simulink model "XMC_FFT2D_HDL_AIE"  (R2021a)
settings: Solver=FixedStepDiscrete  StartTime=0.0  StopTime=256*256*2  RelTol=1e-3
PreLoadFcn:
  | MRIDemo_PreloadFcn;
  | 
  | % configure hardware specifics information
  | clock_frequency = 150e6;
  | 
  | % corner bender info
  | clk = clock_frequency; %Hz
  | Tclk = 1/clk;
  | L2M = 8; % L2M=log2(M)
  | L2N = 8; % L2N=log2(N)
  | M = 2^L2M;
  | N = 2^L2N;
  | SSR = 1;
InitFcn:
  | xlEvaluateHDLBlocks('XMC_FFT2D_HDL_AIE')
undefined symbols (not defined in the file): c, gray, S, vsva2197, xcvc1902
libraries: hdlBasic x138, aieUtilities x3, dspxfrm3 x2, dspsrcs4 x2, aieDSP x2, simulink x1, vmcUtilities x1
(part 2 of 2)

== system XMC_FFT2D_HDL_AIE/hdl_corner_turn/Read BarrelShifter/RotateLeft5 ==
  I : Inport
  Concat : hdlBasic/Concat  num_inputs=2  XmcBlockStatus=1  maskContainerNames=group1  block_type=concat  block_config=sysgen:Concat_config
  Slice : hdlBasic/Slice  nbits=NB  boolean_output=off  mode=Upper Bit Location + Width  bit1=0  base1=MSB of Input  bit0=0  base0=LSB of Input  XmcBlockStatus=1  maskContainerNames=group1  block_type=slice  block_config=sysgen:Slice_config
  Slice1 : hdlBasic/Slice  nbits=W-NB  boolean_output=off  mode=Lower Bit Location + Width  bit1=0  base1=MSB of Input  bit0=0  base0=LSB of Input  XmcBlockStatus=1  maskContainerNames=group1  block_type=slice  block_config=sysgen:Slice_config
  O : Outport
  wires:
  I/1 -> Slice1/1, Slice/1
  Concat/1 -> O/1
  Slice/1 -> Concat/2
  Slice1/1 -> Concat/1

== system XMC_FFT2D_HDL_AIE/hdl_corner_turn/Read BarrelShifter/RotateLeft6 ==
  I : Inport
  Concat : hdlBasic/Concat  num_inputs=2  XmcBlockStatus=1  maskContainerNames=group1  block_type=concat  block_config=sysgen:Concat_config
  Slice : hdlBasic/Slice  nbits=NB  boolean_output=off  mode=Upper Bit Location + Width  bit1=0  base1=MSB of Input  bit0=0  base0=LSB of Input  XmcBlockStatus=1  maskContainerNames=group1  block_type=slice  block_config=sysgen:Slice_config
  Slice1 : hdlBasic/Slice  nbits=W-NB  boolean_output=off  mode=Lower Bit Location + Width  bit1=0  base1=MSB of Input  bit0=0  base0=LSB of Input  XmcBlockStatus=1  maskContainerNames=group1  block_type=slice  block_config=sysgen:Slice_config
  O : Outport
  wires:
  I/1 -> Slice1/1, Slice/1
  Concat/1 -> O/1
  Slice/1 -> Concat/2
  Slice1/1 -> Concat/1

== system XMC_FFT2D_HDL_AIE/hdl_corner_turn/Read BarrelShifter/RotateLeft7 ==
  I : Inport
  Concat : hdlBasic/Concat  num_inputs=2  XmcBlockStatus=1  maskContainerNames=group1  block_type=concat  block_config=sysgen:Concat_config
  Slice : hdlBasic/Slice  nbits=NB  boolean_output=off  mode=Upper Bit Location + Width  bit1=0  base1=MSB of Input  bit0=0  base0=LSB of Input  XmcBlockStatus=1  maskContainerNames=group1  block_type=slice  block_config=sysgen:Slice_config
  Slice1 : hdlBasic/Slice  nbits=W-NB  boolean_output=off  mode=Lower Bit Location + Width  bit1=0  base1=MSB of Input  bit0=0  base0=LSB of Input  XmcBlockStatus=1  maskContainerNames=group1  block_type=slice  block_config=sysgen:Slice_config
  O : Outport
  wires:
  I/1 -> Slice1/1, Slice/1
  Concat/1 -> O/1
  Slice/1 -> Concat/2
  Slice1/1 -> Concat/1

== system XMC_FFT2D_HDL_AIE/hdl_corner_turn/Read BarrelShifter/RotateLeft8 ==
  I : Inport
  Concat : hdlBasic/Concat  num_inputs=2  XmcBlockStatus=1  maskContainerNames=group1  block_type=concat  block_config=sysgen:Concat_config
  Slice : hdlBasic/Slice  nbits=NB  boolean_output=off  mode=Upper Bit Location + Width  bit1=0  base1=MSB of Input  bit0=0  base0=LSB of Input  XmcBlockStatus=1  maskContainerNames=group1  block_type=slice  block_config=sysgen:Slice_config
  Slice1 : hdlBasic/Slice  nbits=W-NB  boolean_output=off  mode=Lower Bit Location + Width  bit1=0  base1=MSB of Input  bit0=0  base0=LSB of Input  XmcBlockStatus=1  maskContainerNames=group1  block_type=slice  block_config=sysgen:Slice_config
  O : Outport
  wires:
  I/1 -> Slice1/1, Slice/1
  Concat/1 -> O/1
  Slice/1 -> Concat/2
  Slice1/1 -> Concat/1

== system XMC_FFT2D_HDL_AIE/hdl_corner_turn/Read BarrelShifter/RotateLeft9 ==
  I : Inport
  Concat : hdlBasic/Concat  num_inputs=2  XmcBlockStatus=1  maskContainerNames=group1  block_type=concat  block_config=sysgen:Concat_config
  Slice : hdlBasic/Slice  nbits=NB  boolean_output=off  mode=Upper Bit Location + Width  bit1=0  base1=MSB of Input  bit0=0  base0=LSB of Input  XmcBlockStatus=1  maskContainerNames=group1  block_type=slice  block_config=sysgen:Slice_config
  Slice1 : hdlBasic/Slice  nbits=W-NB  boolean_output=off  mode=Lower Bit Location + Width  bit1=0  base1=MSB of Input  bit0=0  base0=LSB of Input  XmcBlockStatus=1  maskContainerNames=group1  block_type=slice  block_config=sysgen:Slice_config
  O : Outport
  wires:
  I/1 -> Slice1/1, Slice/1
  Concat/1 -> O/1
  Slice/1 -> Concat/2
  Slice1/1 -> Concat/1

== system XMC_FFT2D_HDL_AIE/hdl_corner_turn/Write BarrelShifter/RotateLeft1 ==
  I : Inport
  Concat : hdlBasic/Concat  num_inputs=2  XmcBlockStatus=1  maskContainerNames=group1  block_type=concat  block_config=sysgen:Concat_config
  Slice : hdlBasic/Slice  nbits=NB  boolean_output=off  mode=Upper Bit Location + Width  bit1=0  base1=MSB of Input  bit0=0  base0=LSB of Input  XmcBlockStatus=1  maskContainerNames=group1  block_type=slice  block_config=sysgen:Slice_config
  Slice1 : hdlBasic/Slice  nbits=W-NB  boolean_output=off  mode=Lower Bit Location + Width  bit1=0  base1=MSB of Input  bit0=0  base0=LSB of Input  XmcBlockStatus=1  maskContainerNames=group1  block_type=slice  block_config=sysgen:Slice_config
  O : Outport
  wires:
  I/1 -> Slice1/1, Slice/1
  Concat/1 -> O/1
  Slice/1 -> Concat/2
  Slice1/1 -> Concat/1

== system XMC_FFT2D_HDL_AIE/hdl_corner_turn/Write BarrelShifter/RotateLeft10 ==
  I : Inport
  Concat : hdlBasic/Concat  num_inputs=2  XmcBlockStatus=1  maskContainerNames=group1  block_type=concat  block_config=sysgen:Concat_config
  Slice : hdlBasic/Slice  nbits=NB  boolean_output=off  mode=Upper Bit Location + Width  bit1=0  base1=MSB of Input  bit0=0  base0=LSB of Input  XmcBlockStatus=1  maskContainerNames=group1  block_type=slice  block_config=sysgen:Slice_config
  Slice1 : hdlBasic/Slice  nbits=W-NB  boolean_output=off  mode=Lower Bit Location + Width  bit1=0  base1=MSB of Input  bit0=0  base0=LSB of Input  XmcBlockStatus=1  maskContainerNames=group1  block_type=slice  block_config=sysgen:Slice_config
  O : Outport
  wires:
  Slice1/1 -> Concat/1
  Slice/1 -> Concat/2
  Concat/1 -> O/1
  I/1 -> Slice/1, Slice1/1

== system XMC_FFT2D_HDL_AIE/hdl_corner_turn/Write BarrelShifter/RotateLeft11 ==
  I : Inport
  Concat : hdlBasic/Concat  num_inputs=2  XmcBlockStatus=1  maskContainerNames=group1  block_type=concat  block_config=sysgen:Concat_config
  Slice : hdlBasic/Slice  nbits=NB  boolean_output=off  mode=Upper Bit Location + Width  bit1=0  base1=MSB of Input  bit0=0  base0=LSB of Input  XmcBlockStatus=1  maskContainerNames=group1  block_type=slice  block_config=sysgen:Slice_config
  Slice1 : hdlBasic/Slice  nbits=W-NB  boolean_output=off  mode=Lower Bit Location + Width  bit1=0  base1=MSB of Input  bit0=0  base0=LSB of Input  XmcBlockStatus=1  maskContainerNames=group1  block_type=slice  block_config=sysgen:Slice_config
  O : Outport
  wires:
  Slice1/1 -> Concat/1
  Slice/1 -> Concat/2
  Concat/1 -> O/1
  I/1 -> Slice/1, Slice1/1

== system XMC_FFT2D_HDL_AIE/hdl_corner_turn/Write BarrelShifter/RotateLeft12 ==
  I : Inport
  Concat : hdlBasic/Concat  num_inputs=2  XmcBlockStatus=1  maskContainerNames=group1  block_type=concat  block_config=sysgen:Concat_config
  Slice : hdlBasic/Slice  nbits=NB  boolean_output=off  mode=Upper Bit Location + Width  bit1=0  base1=MSB of Input  bit0=0  base0=LSB of Input  XmcBlockStatus=1  maskContainerNames=group1  block_type=slice  block_config=sysgen:Slice_config
  Slice1 : hdlBasic/Slice  nbits=W-NB  boolean_output=off  mode=Lower Bit Location + Width  bit1=0  base1=MSB of Input  bit0=0  base0=LSB of Input  XmcBlockStatus=1  maskContainerNames=group1  block_type=slice  block_config=sysgen:Slice_config
  O : Outport
  wires:
  Slice1/1 -> Concat/1
  Slice/1 -> Concat/2
  Concat/1 -> O/1
  I/1 -> Slice/1, Slice1/1

== system XMC_FFT2D_HDL_AIE/hdl_corner_turn/Write BarrelShifter/RotateLeft13 ==
  I : Inport
  Concat : hdlBasic/Concat  num_inputs=2  XmcBlockStatus=1  maskContainerNames=group1  block_type=concat  block_config=sysgen:Concat_config
  Slice : hdlBasic/Slice  nbits=NB  boolean_output=off  mode=Upper Bit Location + Width  bit1=0  base1=MSB of Input  bit0=0  base0=LSB of Input  XmcBlockStatus=1  maskContainerNames=group1  block_type=slice  block_config=sysgen:Slice_config
  Slice1 : hdlBasic/Slice  nbits=W-NB  boolean_output=off  mode=Lower Bit Location + Width  bit1=0  base1=MSB of Input  bit0=0  base0=LSB of Input  XmcBlockStatus=1  maskContainerNames=group1  block_type=slice  block_config=sysgen:Slice_config
  O : Outport
  wires:
  Slice1/1 -> Concat/1
  Slice/1 -> Concat/2
  Concat/1 -> O/1
  I/1 -> Slice/1, Slice1/1

== system XMC_FFT2D_HDL_AIE/hdl_corner_turn/Write BarrelShifter/RotateLeft14 ==
  I : Inport
  Concat : hdlBasic/Concat  num_inputs=2  XmcBlockStatus=1  maskContainerNames=group1  block_type=concat  block_config=sysgen:Concat_config
  Slice : hdlBasic/Slice  nbits=NB  boolean_output=off  mode=Upper Bit Location + Width  bit1=0  base1=MSB of Input  bit0=0  base0=LSB of Input  XmcBlockStatus=1  maskContainerNames=group1  block_type=slice  block_config=sysgen:Slice_config
  Slice1 : hdlBasic/Slice  nbits=W-NB  boolean_output=off  mode=Lower Bit Location + Width  bit1=0  base1=MSB of Input  bit0=0  base0=LSB of Input  XmcBlockStatus=1  maskContainerNames=group1  block_type=slice  block_config=sysgen:Slice_config
  O : Outport
  wires:
  Slice1/1 -> Concat/1
  Slice/1 -> Concat/2
  Concat/1 -> O/1
  I/1 -> Slice/1, Slice1/1

== system XMC_FFT2D_HDL_AIE/hdl_corner_turn/Write BarrelShifter/RotateLeft15 ==
  I : Inport
  Concat : hdlBasic/Concat  num_inputs=2  XmcBlockStatus=1  maskContainerNames=group1  block_type=concat  block_config=sysgen:Concat_config
  Slice : hdlBasic/Slice  nbits=NB  boolean_output=off  mode=Upper Bit Location + Width  bit1=0  base1=MSB of Input  bit0=0  base0=LSB of Input  XmcBlockStatus=1  maskContainerNames=group1  block_type=slice  block_config=sysgen:Slice_config
  Slice1 : hdlBasic/Slice  nbits=W-NB  boolean_output=off  mode=Lower Bit Location + Width  bit1=0  base1=MSB of Input  bit0=0  base0=LSB of Input  XmcBlockStatus=1  maskContainerNames=group1  block_type=slice  block_config=sysgen:Slice_config
  O : Outport
  wires:
  Slice1/1 -> Concat/1
  Slice/1 -> Concat/2
  Concat/1 -> O/1
  I/1 -> Slice/1, Slice1/1

== system XMC_FFT2D_HDL_AIE/hdl_corner_turn/Write BarrelShifter/RotateLeft2 ==
  I : Inport
  Concat : hdlBasic/Concat  num_inputs=2  XmcBlockStatus=1  maskContainerNames=group1  block_type=concat  block_config=sysgen:Concat_config
  Slice : hdlBasic/Slice  nbits=NB  boolean_output=off  mode=Upper Bit Location + Width  bit1=0  base1=MSB of Input  bit0=0  base0=LSB of Input  XmcBlockStatus=1  maskContainerNames=group1  block_type=slice  block_config=sysgen:Slice_config
  Slice1 : hdlBasic/Slice  nbits=W-NB  boolean_output=off  mode=Lower Bit Location + Width  bit1=0  base1=MSB of Input  bit0=0  base0=LSB of Input  XmcBlockStatus=1  maskContainerNames=group1  block_type=slice  block_config=sysgen:Slice_config
  O : Outport
  wires:
  Slice1/1 -> Concat/1
  Slice/1 -> Concat/2
  Concat/1 -> O/1
  I/1 -> Slice/1, Slice1/1

== system XMC_FFT2D_HDL_AIE/hdl_corner_turn/Write BarrelShifter/RotateLeft3 ==
  I : Inport
  Concat : hdlBasic/Concat  num_inputs=2  XmcBlockStatus=1  maskContainerNames=group1  block_type=concat  block_config=sysgen:Concat_config
  Slice : hdlBasic/Slice  nbits=NB  boolean_output=off  mode=Upper Bit Location + Width  bit1=0  base1=MSB of Input  bit0=0  base0=LSB of Input  XmcBlockStatus=1  maskContainerNames=group1  block_type=slice  block_config=sysgen:Slice_config
  Slice1 : hdlBasic/Slice  nbits=W-NB  boolean_output=off  mode=Lower Bit Location + Width  bit1=0  base1=MSB of Input  bit0=0  base0=LSB of Input  XmcBlockStatus=1  maskContainerNames=group1  block_type=slice  block_config=sysgen:Slice_config
  O : Outport
  wires:
  Slice1/1 -> Concat/1
  Slice/1 -> Concat/2
  Concat/1 -> O/1
  I/1 -> Slice/1, Slice1/1

== system XMC_FFT2D_HDL_AIE/hdl_corner_turn/Write BarrelShifter/RotateLeft4 ==
  I : Inport
  Concat : hdlBasic/Concat  num_inputs=2  XmcBlockStatus=1  maskContainerNames=group1  block_type=concat  block_config=sysgen:Concat_config
  Slice : hdlBasic/Slice  nbits=NB  boolean_output=off  mode=Upper Bit Location + Width  bit1=0  base1=MSB of Input  bit0=0  base0=LSB of Input  XmcBlockStatus=1  maskContainerNames=group1  block_type=slice  block_config=sysgen:Slice_config
  Slice1 : hdlBasic/Slice  nbits=W-NB  boolean_output=off  mode=Lower Bit Location + Width  bit1=0  base1=MSB of Input  bit0=0  base0=LSB of Input  XmcBlockStatus=1  maskContainerNames=group1  block_type=slice  block_config=sysgen:Slice_config
  O : Outport
  wires:
  Slice1/1 -> Concat/1
  Slice/1 -> Concat/2
  Concat/1 -> O/1
  I/1 -> Slice/1, Slice1/1

== system XMC_FFT2D_HDL_AIE/hdl_corner_turn/Write BarrelShifter/RotateLeft5 ==
  I : Inport
  Concat : hdlBasic/Concat  num_inputs=2  XmcBlockStatus=1  maskContainerNames=group1  block_type=concat  block_config=sysgen:Concat_config
  Slice : hdlBasic/Slice  nbits=NB  boolean_output=off  mode=Upper Bit Location + Width  bit1=0  base1=MSB of Input  bit0=0  base0=LSB of Input  XmcBlockStatus=1  maskContainerNames=group1  block_type=slice  block_config=sysgen:Slice_config
  Slice1 : hdlBasic/Slice  nbits=W-NB  boolean_output=off  mode=Lower Bit Location + Width  bit1=0  base1=MSB of Input  bit0=0  base0=LSB of Input  XmcBlockStatus=1  maskContainerNames=group1  block_type=slice  block_config=sysgen:Slice_config
  O : Outport
  wires:
  Slice1/1 -> Concat/1
  Slice/1 -> Concat/2
  Concat/1 -> O/1
  I/1 -> Slice/1, Slice1/1

== system XMC_FFT2D_HDL_AIE/hdl_corner_turn/Write BarrelShifter/RotateLeft6 ==
  I : Inport
  Concat : hdlBasic/Concat  num_inputs=2  XmcBlockStatus=1  maskContainerNames=group1  block_type=concat  block_config=sysgen:Concat_config
  Slice : hdlBasic/Slice  nbits=NB  boolean_output=off  mode=Upper Bit Location + Width  bit1=0  base1=MSB of Input  bit0=0  base0=LSB of Input  XmcBlockStatus=1  maskContainerNames=group1  block_type=slice  block_config=sysgen:Slice_config
  Slice1 : hdlBasic/Slice  nbits=W-NB  boolean_output=off  mode=Lower Bit Location + Width  bit1=0  base1=MSB of Input  bit0=0  base0=LSB of Input  XmcBlockStatus=1  maskContainerNames=group1  block_type=slice  block_config=sysgen:Slice_config
  O : Outport
  wires:
  Slice1/1 -> Concat/1
  Slice/1 -> Concat/2
  Concat/1 -> O/1
  I/1 -> Slice/1, Slice1/1

== system XMC_FFT2D_HDL_AIE/hdl_corner_turn/Write BarrelShifter/RotateLeft7 ==
  I : Inport
  Concat : hdlBasic/Concat  num_inputs=2  XmcBlockStatus=1  maskContainerNames=group1  block_type=concat  block_config=sysgen:Concat_config
  Slice : hdlBasic/Slice  nbits=NB  boolean_output=off  mode=Upper Bit Location + Width  bit1=0  base1=MSB of Input  bit0=0  base0=LSB of Input  XmcBlockStatus=1  maskContainerNames=group1  block_type=slice  block_config=sysgen:Slice_config
  Slice1 : hdlBasic/Slice  nbits=W-NB  boolean_output=off  mode=Lower Bit Location + Width  bit1=0  base1=MSB of Input  bit0=0  base0=LSB of Input  XmcBlockStatus=1  maskContainerNames=group1  block_type=slice  block_config=sysgen:Slice_config
  O : Outport
  wires:
  Slice1/1 -> Concat/1
  Slice/1 -> Concat/2
  Concat/1 -> O/1
  I/1 -> Slice/1, Slice1/1

== system XMC_FFT2D_HDL_AIE/hdl_corner_turn/Write BarrelShifter/RotateLeft8 ==
  I : Inport
  Concat : hdlBasic/Concat  num_inputs=2  XmcBlockStatus=1  maskContainerNames=group1  block_type=concat  block_config=sysgen:Concat_config
  Slice : hdlBasic/Slice  nbits=NB  boolean_output=off  mode=Upper Bit Location + Width  bit1=0  base1=MSB of Input  bit0=0  base0=LSB of Input  XmcBlockStatus=1  maskContainerNames=group1  block_type=slice  block_config=sysgen:Slice_config
  Slice1 : hdlBasic/Slice  nbits=W-NB  boolean_output=off  mode=Lower Bit Location + Width  bit1=0  base1=MSB of Input  bit0=0  base0=LSB of Input  XmcBlockStatus=1  maskContainerNames=group1  block_type=slice  block_config=sysgen:Slice_config
  O : Outport
  wires:
  Slice1/1 -> Concat/1
  Slice/1 -> Concat/2
  Concat/1 -> O/1
  I/1 -> Slice/1, Slice1/1

== system XMC_FFT2D_HDL_AIE/hdl_corner_turn/Write BarrelShifter/RotateLeft9 ==
  I : Inport
  Concat : hdlBasic/Concat  num_inputs=2  XmcBlockStatus=1  maskContainerNames=group1  block_type=concat  block_config=sysgen:Concat_config
  Slice : hdlBasic/Slice  nbits=NB  boolean_output=off  mode=Upper Bit Location + Width  bit1=0  base1=MSB of Input  bit0=0  base0=LSB of Input  XmcBlockStatus=1  maskContainerNames=group1  block_type=slice  block_config=sysgen:Slice_config
  Slice1 : hdlBasic/Slice  nbits=W-NB  boolean_output=off  mode=Lower Bit Location + Width  bit1=0  base1=MSB of Input  bit0=0  base0=LSB of Input  XmcBlockStatus=1  maskContainerNames=group1  block_type=slice  block_config=sysgen:Slice_config
  O : Outport
  wires:
  Slice1/1 -> Concat/1
  Slice/1 -> Concat/2
  Concat/1 -> O/1
  I/1 -> Slice/1, Slice1/1
